simulink model "mm"  (R2016a)
settings: Solver=VariableStepAuto  StartTime=0.0  StopTime=120.0  RelTol=1e-3
libraries: simulink x1
settings Model: Creator=Marcelo  LastModifiedBy=Marcelo

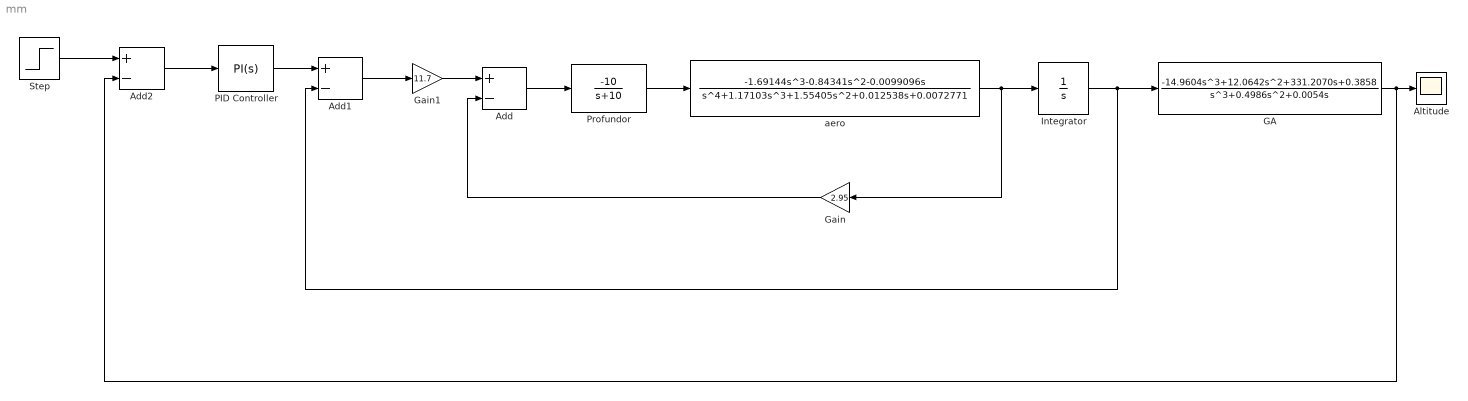
== system mm ==
  Add : Sum  Inputs=+-
  Add1 : Sum  Inputs=+-
  Add2 : Sum  Inputs=+-
  Altitude : Scope
  GA : TransferFcn  Numerator=[-14.9604 12.0642 331.2070 0.3858]  Denominator="[1 0.4986    0.0054         0]"
  Gain : Gain  Gain=2.95
  Gain1 : Gain  Gain=11.7
  Integrator : Integrator
  PID Controller : simulink/Continuous/PID Controller  Controller=PI  TimeDomain=Continuous-time  SampleTime=-1  IntegratorMethod=Forward Euler  FilterMethod=Forward Euler  Form=Parallel  UseFilter=on  ControllerParametersSource=internal  P=0.000674  I=4.28e-06  D=0  N=100  InitialConditionSource=internal  InitialConditionForIntegrator=0  InitialConditionForFilter=0  ExternalReset=none  LimitOutput=off  UpperSaturationLimit=inf  LowerSaturationLimit=-inf  LinearizeAsGain=on  AntiWindupMode=none  Kb=1  TrackingMode=off  Kt=1  PParamMin=[]  PParamMax=[]  IParamMin=[]  IParamMax=[]  DParamMin=[]  DParamMax=[]  NParamMin=[]  NParamMax=[]  KbParamMin=[]  KbParamMax=[]  KtParamMin=[]  KtParamMax=[]  POutMin=[]  POutMax=[]  IOutMin=[]  IOutMax=[]  DOutMin=[]  DOutMax=[]  NOutMin=[]  NOutMax=[]  KbOutMin=[]  KbOutMax=[]  KtOutMin=[]  KtOutMax=[]  IntegratorOutMin=[]  IntegratorOutMax=[]  FilterOutMin=[]  FilterOutMax=[]  SumOutMin=[]  SumOutMax=[]  SumI1OutMin=[]  SumI1OutMax=[]  SumI2OutMin=[]  SumI2OutMax=[]  SumI3OutMin=[]  SumI3OutMax=[]  SumDOutMin=[]  SumDOutMax=[]  SaturationOutMin=[]  SaturationOutMax=[]  IntegratorContinuousStateAttributes=''  IntegratorStateMustResolveToSignalObject=off  IntegratorRTWStateStorageClass=Auto  FilterContinuousStateAttributes=''  FilterStateMustResolveToSignalObject=off  FilterRTWStateStorageClass=Auto  DifferentiatorICPrevScaledInput=0  DifferentiatorOutMin=[]  DifferentiatorOutMax=[]
  Profundor : TransferFcn  Numerator=[-10]  Denominator=[1 10]
  Step : Step  Time=20  After=1000  SampleTime=0
  aero : TransferFcn  Numerator=[-1.69144 -0.84341 -0.0099096 0]  Denominator=[1 1.17103 1.55405 0.012538 0.0072771]
  wires:
  aero/1 -> Gain/1, Integrator/1
  Profundor/1 -> aero/1
  Add/1 -> Profundor/1
  Gain/1 -> Add/2
  Gain1/1 -> Add/1
  Add1/1 -> Gain1/1
  Integrator/1 -> GA/1, Add1/2
  GA/1 -> Add2/2, Altitude/1
  Add2/1 -> PID Controller/1
  Step/1 -> Add2/1
  PID Controller/1 -> Add1/1
